simulink model "untitled1"  (R2022b)
settings: Solver=FixedStepAuto  StartTime=0.0  StopTime=10.0  FixedStep=0.1  RelTol=1e-3  EnableMultiTasking=on
settings Model: Creator=mluser  LastModifiedBy=mluser
settings SolverCC: AlgebraicLoopSolver=TrustRegion  AutoInsertRateTranBlk=on
settings DataIOCC: LimitDataPoints=on
settings OptimizationCC: LifeSpan=inf
settings DebuggingCC: UnconnectedInputMsg=warning  UnconnectedOutputMsg=warning  UnconnectedLineMsg=warning  AllowSymbolicDim=off  SFUnexpectedBacktrackingDiag=warning  SFNoUnconditionalDefaultTransitionDiag=warning  SFExecutionAtInitializationDiag=none  ArithmeticOperatorsInVariantConditions=warning
settings ModelReferenceCC: EnableRefExpFcnMdlSchedulingChecks=on
settings SFSimCC: SimUseLocalCustomCode=off  CustomCodeUndefinedFunction=UseInterfaceOnly
settings RTWCC: RTWUseLocalCustomCode=off  DLArmComputeVersion=19.05
settings CodeAppCC: StateflowObjectComments=on
settings GRTTargetCC: TargetLangStandard=C89/C90 (ANSI)
settings ConfigComp: CovMetricSettings=dw  CovSaveCumulativeToWorkspaceVar=on  CovSaveSingleToWorkspaceVar=on  CovExternalEMLEnable=off

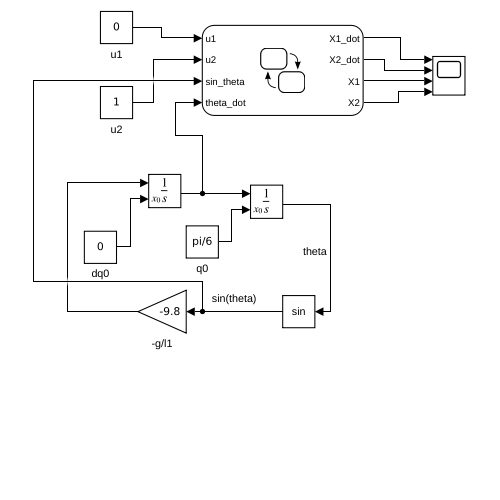
[thumbnail: Simulink's stored preview of the top-level diagram]
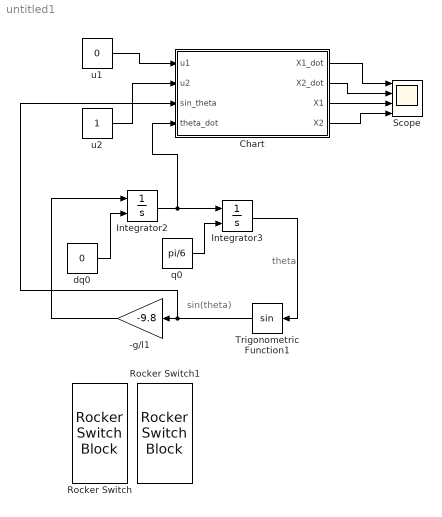
== system untitled1 ==
  note: sin(theta)
  note: theta
  -g/l1 : Gain  Gain=-9.8
  Chart : Stateflow chart  TreatAsAtomicUnit=on
  Integrator2 : Integrator  InitialConditionSource=external
  Integrator3 : Integrator  InitialConditionSource=external
  Rocker Switch : RockerSwitchBlock
      settings: Values={{'Off', 'On'}, [0 1]}
  Rocker Switch1 : RockerSwitchBlock
      settings: Values={{'Off', 'On'}, [0 1]}
  Scope : Scope  NumInputPorts=4
  Trigonometric Function1 : Trigonometry
  dq0 : Constant  Value=0
  q0 : Constant  Value=pi/6
  u1 : Constant  Value=0
  u2 : Constant
  wires:
  Chart/1(X1_dot) -> Scope/1
  Chart/2(X2_dot) -> Scope/2
  u1/1 -> Chart/1(u1)
  u2/1 -> Chart/2(u2)
  Chart/3(X1) -> Scope/3
  Chart/4(X2) -> Scope/4
  q0/1 -> Integrator3/2
  Integrator3/1 -> Trigonometric Function1/1
  Integrator2/1 -> Chart/4(theta_dot), Integrator3/1
  -g/l1/1 -> Integrator2/1
  dq0/1 -> Integrator2/2
  Trigonometric Function1/1 -> Chart/3(sin_theta), -g/l1/1

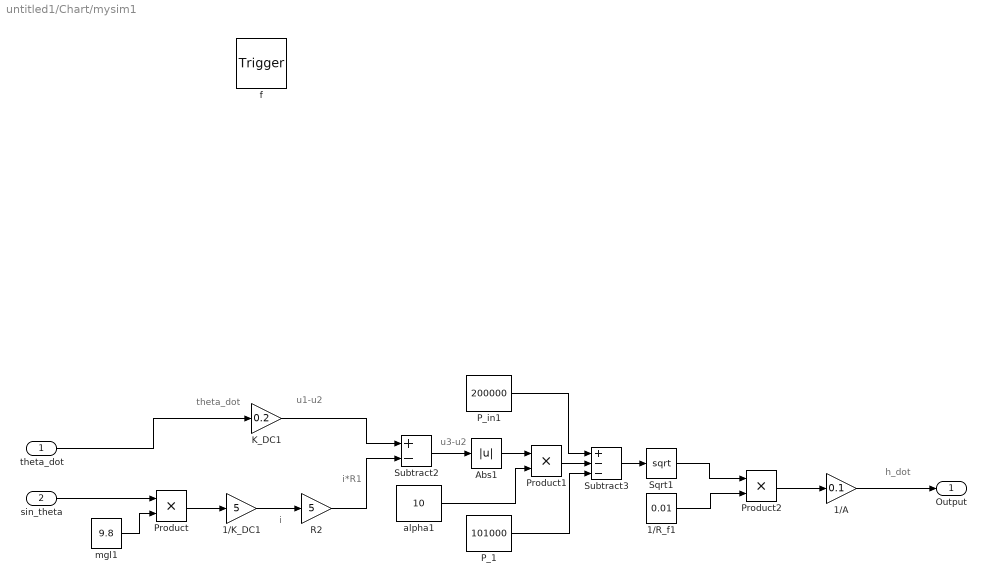
== system untitled1/Chart/mysim1 ==
  note: u3-u2
  note: h_dot
  note: u1-u2
  note: i
  note: theta_dot
  note: i*R1
  theta_dot : Inport  OutDataTypeStr=double  PortDimensions=1
  sin_theta : Inport  Port=2  OutDataTypeStr=double  PortDimensions=1
  f : TriggerPort  TriggerType=function-call  VariantControl=(inherit)
      settings: CopyFcn=Stateflow.SLINSF.SimulinkMan.removeBlockPreDeleteFcn  PreDeleteFcn=Stateflow.SLINSF.SimulinkMan.unsafePredeleteFcn
  1/A : Gain  Gain=0.1
  1/K_DC1 : Gain  Gain=5
  1/R_f1 : Constant  Value=0.01
  Abs1 : Abs  SaturateOnIntegerOverflow=off
  K_DC1 : Gain  Gain=0.2
  P_1 : Constant  Value=101000
  P_in1 : Constant  Value=200000
  Product : Product
  Product1 : Product
  Product2 : Product
  R2 : Gain  Gain=5
  Sqrt1 : Sqrt
  Subtract2 : Sum  Inputs=+-
  Subtract3 : Sum  Inputs=+--
  alpha1 : Constant  Value=10
  mgl1 : Constant  Value=9.8
  Output : Outport
  wires:
  P_1/1 -> Subtract3/3
  Product1/1 -> Subtract3/2
  1/K_DC1/1 -> R2/1
  Subtract3/1 -> Sqrt1/1
  alpha1/1 -> Product1/2
  Subtract2/1 -> Abs1/1
  1/R_f1/1 -> Product2/2
  P_in1/1 -> Subtract3/1
  K_DC1/1 -> Subtract2/1
  Sqrt1/1 -> Product2/1
  Abs1/1 -> Product1/1
  Product/1 -> 1/K_DC1/1
  mgl1/1 -> Product/2
  R2/1 -> Subtract2/2
  Product2/1 -> 1/A/1
  1/A/1 -> Output/1
  theta_dot/1 -> K_DC1/1
  sin_theta/1 -> Product/1

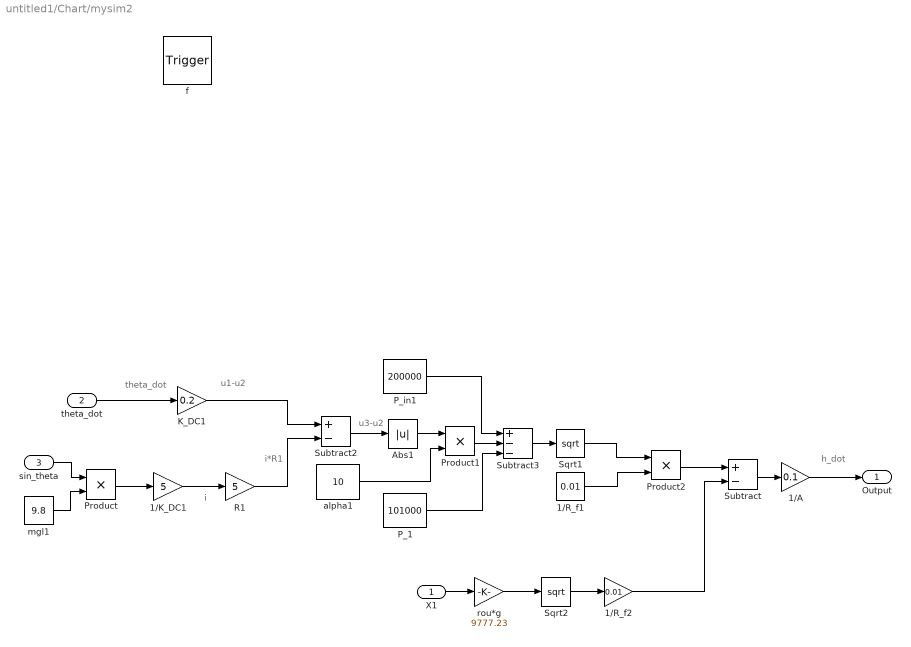
== system untitled1/Chart/mysim2 ==
  note: u3-u2
  note: h_dot
  note: u1-u2
  note: i
  note: theta_dot
  note: i*R1
  X1 : Inport  OutDataTypeStr=double  PortDimensions=1
  theta_dot : Inport  Port=2  OutDataTypeStr=double  PortDimensions=1
  sin_theta : Inport  Port=3  OutDataTypeStr=double  PortDimensions=1
  f : TriggerPort  TriggerType=function-call  VariantControl=(inherit)
      settings: CopyFcn=Stateflow.SLINSF.SimulinkMan.removeBlockPreDeleteFcn  PreDeleteFcn=Stateflow.SLINSF.SimulinkMan.unsafePredeleteFcn
  1/A : Gain  Gain=0.1
  1/K_DC1 : Gain  Gain=5
  1/R_f1 : Constant  Value=0.01
  1/R_f2 : Gain  Gain=0.01
  Abs1 : Abs  SaturateOnIntegerOverflow=off
  K_DC1 : Gain  Gain=0.2
  P_1 : Constant  Value=101000
  P_in1 : Constant  Value=200000
  Product : Product
  Product1 : Product
  Product2 : Product
  R1 : Gain  Gain=5
  Sqrt1 : Sqrt
  Sqrt2 : Sqrt
  Subtract : Sum  Inputs=+-
  Subtract2 : Sum  Inputs=+-
  Subtract3 : Sum  Inputs=+--
  alpha1 : Constant  Value=10
  mgl1 : Constant  Value=9.8
  rou*g : Gain  Gain=9777.23
  Output : Outport
  wires:
  P_1/1 -> Subtract3/3
  Product1/1 -> Subtract3/2
  1/K_DC1/1 -> R1/1
  Subtract3/1 -> Sqrt1/1
  alpha1/1 -> Product1/2
  Subtract2/1 -> Abs1/1
  1/R_f1/1 -> Product2/2
  P_in1/1 -> Subtract3/1
  K_DC1/1 -> Subtract2/1
  Sqrt1/1 -> Product2/1
  Abs1/1 -> Product1/1
  Product/1 -> 1/K_DC1/1
  mgl1/1 -> Product/2
  R1/1 -> Subtract2/2
  Product2/1 -> Subtract/1
  Subtract/1 -> 1/A/1
  1/A/1 -> Output/1
  X1/1 -> rou*g/1
  rou*g/1 -> Sqrt2/1
  Sqrt2/1 -> 1/R_f2/1
  1/R_f2/1 -> Subtract/2
  theta_dot/1 -> K_DC1/1
  sin_theta/1 -> Product/1

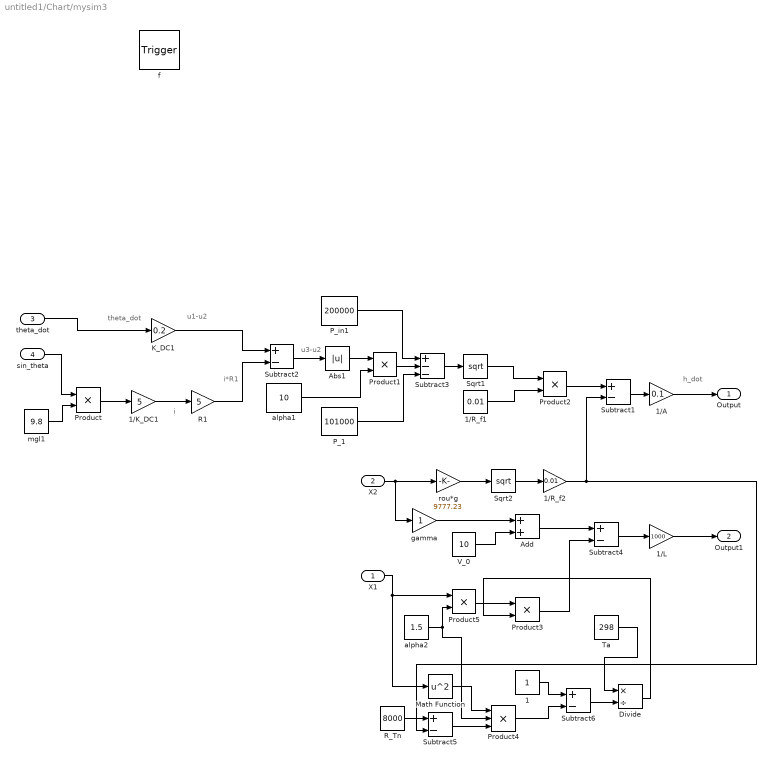
== system untitled1/Chart/mysim3 ==
  note: u3-u2
  note: h_dot
  note: u1-u2
  note: i
  note: theta_dot
  note: i*R1
  X1 : Inport  OutDataTypeStr=double  PortDimensions=1
  X2 : Inport  Port=2  OutDataTypeStr=double  PortDimensions=1
  theta_dot : Inport  Port=3  OutDataTypeStr=double  PortDimensions=1
  sin_theta : Inport  Port=4  OutDataTypeStr=double  PortDimensions=1
  f : TriggerPort  TriggerType=function-call  VariantControl=(inherit)
      settings: CopyFcn=Stateflow.SLINSF.SimulinkMan.removeBlockPreDeleteFcn  PreDeleteFcn=Stateflow.SLINSF.SimulinkMan.unsafePredeleteFcn
  1 : Constant
  1/A : Gain  Gain=0.1
  1/K_DC1 : Gain  Gain=5
  1/L : Gain  Gain=1000
  1/R_f1 : Constant  Value=0.01
  1/R_f2 : Gain  Gain=0.01
  Abs1 : Abs  SaturateOnIntegerOverflow=off
  Add : Sum
  Divide : Product  Inputs=*/
  K_DC1 : Gain  Gain=0.2
  Math Function : Math  Operator=square
  P_1 : Constant  Value=101000
  P_in1 : Constant  Value=200000
  Product{,1..3,5} (5 alike) : Product
  Product4 : Product  Inputs=3
  R1 : Gain  Gain=5
  R_Tn : Constant  Value=8000
  Sqrt1 : Sqrt
  Sqrt2 : Sqrt
  Subtract{1..2,4..6} (5 alike) : Sum  Inputs=+-
  Subtract3 : Sum  Inputs=+--
  Ta : Constant  Value=298
  V_0 : Constant  Value=10
  alpha1 : Constant  Value=10
  alpha2 : Constant  Value=1.5
  gamma : Gain
  mgl1 : Constant  Value=9.8
  rou*g : Gain  Gain=9777.23
  Output : Outport
  Output1 : Outport  Port=2
  wires:
  P_1/1 -> Subtract3/3
  Product1/1 -> Subtract3/2
  1/K_DC1/1 -> R1/1
  Subtract3/1 -> Sqrt1/1
  alpha1/1 -> Product1/2
  Subtract2/1 -> Abs1/1
  1/R_f1/1 -> Product2/2
  P_in1/1 -> Subtract3/1
  K_DC1/1 -> Subtract2/1
  Sqrt1/1 -> Product2/1
  Abs1/1 -> Product1/1
  Product/1 -> 1/K_DC1/1
  mgl1/1 -> Product/2
  R1/1 -> Subtract2/2
  Product2/1 -> Subtract1/1
  Subtract1/1 -> 1/A/1
  1/A/1 -> Output/1
  X2/1 -> gamma/1, rou*g/1
  rou*g/1 -> Sqrt2/1
  Sqrt2/1 -> 1/R_f2/1
  1/R_f2/1 -> Subtract1/2, Subtract5/2
  gamma/1 -> Add/1
  V_0/1 -> Add/2
  Product5/1 -> Product3/1
  Add/1 -> Subtract4/1
  Product3/1 -> Subtract4/2
  Subtract4/1 -> 1/L/1
  1/L/1 -> Output1/1
  Math Function/1 -> Product4/1
  alpha2/1 -> Product5/2, Product4/2
  X1/1 -> Math Function/1, Product5/1
  Subtract5/1 -> Product4/3
  R_Tn/1 -> Subtract5/1
  Product4/1 -> Subtract6/2
  1/1 -> Subtract6/1
  Subtract6/1 -> Divide/2
  Ta/1 -> Divide/1
  Divide/1 -> Product3/2
  theta_dot/1 -> K_DC1/1
  sin_theta/1 -> Product/1

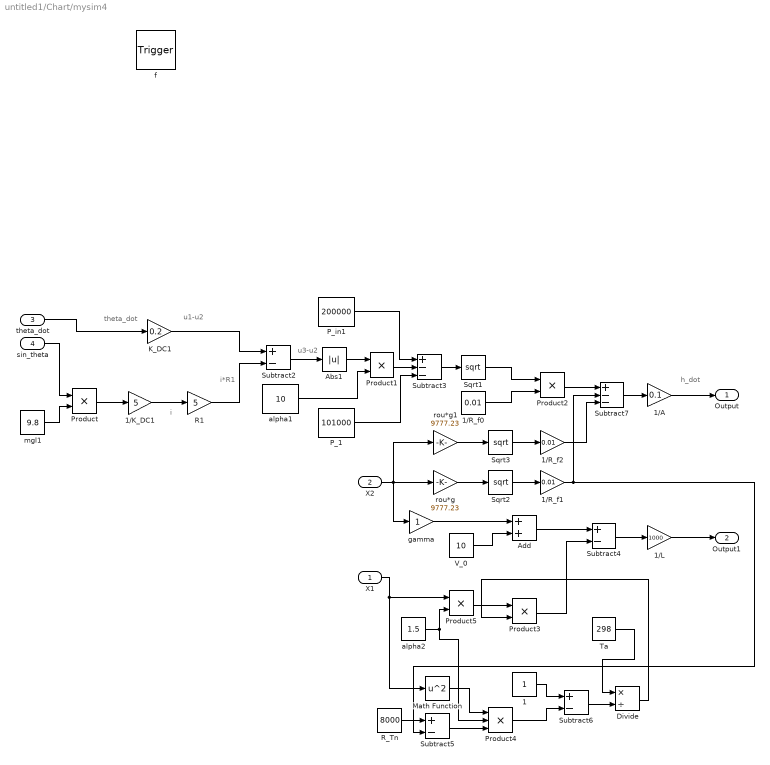
== system untitled1/Chart/mysim4 ==
  note: u3-u2
  note: h_dot
  note: u1-u2
  note: i
  note: theta_dot
  note: i*R1
  X1 : Inport  OutDataTypeStr=double  PortDimensions=1
  X2 : Inport  Port=2  OutDataTypeStr=double  PortDimensions=1
  theta_dot : Inport  Port=3  OutDataTypeStr=double  PortDimensions=1
  sin_theta : Inport  Port=4  OutDataTypeStr=double  PortDimensions=1
  f : TriggerPort  TriggerType=function-call  VariantControl=(inherit)
      settings: CopyFcn=Stateflow.SLINSF.SimulinkMan.removeBlockPreDeleteFcn  PreDeleteFcn=Stateflow.SLINSF.SimulinkMan.unsafePredeleteFcn
  1 : Constant
  1/A : Gain  Gain=0.1
  1/K_DC1 : Gain  Gain=5
  1/L : Gain  Gain=1000
  1/R_f0 : Constant  Value=0.01
  1/R_f1 : Gain  Gain=0.01
  1/R_f2 : Gain  Gain=0.01
  Abs1 : Abs  SaturateOnIntegerOverflow=off
  Add : Sum
  Divide : Product  Inputs=*/
  K_DC1 : Gain  Gain=0.2
  Math Function : Math  Operator=square
  P_1 : Constant  Value=101000
  P_in1 : Constant  Value=200000
  Product{,1..3,5} (5 alike) : Product
  Product4 : Product  Inputs=3
  R1 : Gain  Gain=5
  R_Tn : Constant  Value=8000
  Sqrt1 : Sqrt
  Sqrt2 : Sqrt
  Sqrt3 : Sqrt
  Subtract{2,4..6} (4 alike) : Sum  Inputs=+-
  Subtract3 : Sum  Inputs=+--
  Subtract7 : Sum  Inputs=+--
  Ta : Constant  Value=298
  V_0 : Constant  Value=10
  alpha1 : Constant  Value=10
  alpha2 : Constant  Value=1.5
  gamma : Gain
  mgl1 : Constant  Value=9.8
  rou*g : Gain  Gain=9777.23
  rou*g1 : Gain  Gain=9777.23
  Output : Outport
  Output1 : Outport  Port=2
  wires:
  P_1/1 -> Subtract3/3
  Product1/1 -> Subtract3/2
  1/K_DC1/1 -> R1/1
  Subtract3/1 -> Sqrt1/1
  alpha1/1 -> Product1/2
  Subtract2/1 -> Abs1/1
  1/R_f0/1 -> Product2/2
  P_in1/1 -> Subtract3/1
  K_DC1/1 -> Subtract2/1
  Sqrt1/1 -> Product2/1
  Abs1/1 -> Product1/1
  Product/1 -> 1/K_DC1/1
  mgl1/1 -> Product/2
  R1/1 -> Subtract2/2
  Subtract7/1 -> 1/A/1
  1/A/1 -> Output/1
  X2/1 -> rou*g1/1, gamma/1, rou*g/1
  rou*g/1 -> Sqrt2/1
  Sqrt2/1 -> 1/R_f1/1
  1/R_f1/1 -> Subtract5/2, Subtract7/2
  gamma/1 -> Add/1
  V_0/1 -> Add/2
  Product5/1 -> Product3/1
  Add/1 -> Subtract4/1
  Product3/1 -> Subtract4/2
  Subtract4/1 -> 1/L/1
  1/L/1 -> Output1/1
  Math Function/1 -> Product4/1
  alpha2/1 -> Product5/2, Product4/2
  X1/1 -> Math Function/1, Product5/1
  Subtract5/1 -> Product4/3
  R_Tn/1 -> Subtract5/1
  Product4/1 -> Subtract6/2
  1/1 -> Subtract6/1
  Subtract6/1 -> Divide/2
  Ta/1 -> Divide/1
  Divide/1 -> Product3/2
  Product2/1 -> Subtract7/1
  rou*g1/1 -> Sqrt3/1
  Sqrt3/1 -> 1/R_f2/1
  1/R_f2/1 -> Subtract7/3
  theta_dot/1 -> K_DC1/1
  sin_theta/1 -> Product/1

== stateflow chart untitled1/Chart ==
  state State2
    entry:
    X1=r;
    X1_dot=mysim2(X1,theta_dot,sin_theta);
    X2_dot=0;
  state State1 %State Name
    entry:
    X1=r;
    X1_dot=mysim1(theta_dot,sin_theta);
    X2_dot=0;
  state Output = mysim1(theta_dot,sin_theta) [function]
  state State4 %State Name
    entry:
    X1=r;
    [Output,Output1]=mysim4(X1,X2,theta_dot,sin_theta);
    X1_dot=Output;
    X2_dot=Output1;
  state State3 %State Name
    entry:
    X1=r;
    [Output,Output1]=mysim3(X1,X2,theta_dot,sin_theta);
    X1_dot=Output;
    X2_dot=Output1;
  state Output = mysim2(X1,theta_dot,sin_theta) [function]
  state [Output,Output1] = mysim3(X1,X2,theta_dot,sin_theta) [function]
  state [Output,Output1] = mysim4(X1,X2,theta_dot,sin_theta) [function]
  (default) -> State1 %State Name : {X1=0;
      | X2=0;}
  State1 %State Name -> State2 [order 1] : [u1== 0&&u2==1]
      | % [transition condition]{action}
  State1 %State Name -> State4 %State Name [order 3] : [u1== 1&&u2==1]
  State2 -> State1 %State Name [order 1] : [u1== 0&&u2==0]
  State3 %State Name -> State2 [order 3] : [u1== 0&&u2==1]
  State2 -> State3 %State Name [order 3] : [u1== 1&&u2==0]
  State2 -> State4 %State Name [order 2] : [u1== 1&&u2==1]
  State4 %State Name -> State2 [order 1] : [u1==0&&u2==1]
  State1 %State Name -> State3 %State Name [order 2] : [u1== 1&&u2==0]
  State3 %State Name -> State1 %State Name [order 1] : [u1== 0&&u2==0]
  State4 %State Name -> State1 %State Name [order 3] : [u1== 0&&u2==0]
  State3 %State Name -> State4 %State Name [order 2] : [u1== 1&&u2==1]
  State4 %State Name -> State3 %State Name [order 2] : [u1== 1&&u2==0]
  data: Output function_output; theta_dot function_input double size=1; sin_theta function_input double size=1; Output function_output; X1 function_input double size=1; theta_dot function_input double size=1; sin_theta function_input double size=1; X1 function_input double size=1; Output function_output; X2 function_input double size=1; Output1 function_output; theta_dot function_input double size=1; sin_theta function_input double size=1; X1 function_input double size=1; Output function_output; X2 function_input double size=1; Output1 function_output; theta_dot function_input double size=1; sin_theta function_input double size=1; X1_dot output; X2_dot output; Output local; Output1 local; u1 input; u2 input; X1 output; X2 output; sin_theta input; theta_dot input
